simulink model "que2"  (R2023a)
settings: Solver=VariableStepAuto  StartTime=0.0  StopTime=500  RelTol=1e-3
settings Model: Creator=Hasee  LastModifiedBy=Administrator

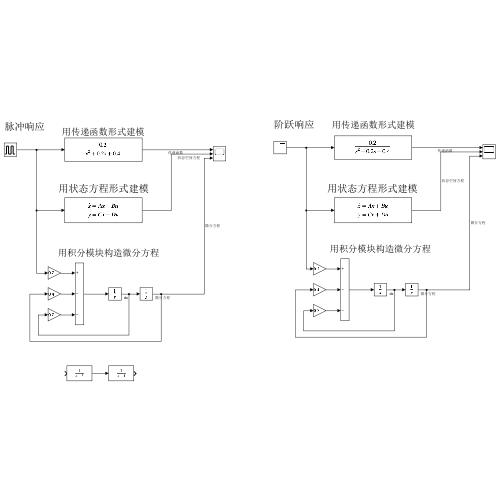
[thumbnail: Simulink's stored preview of the top-level diagram]
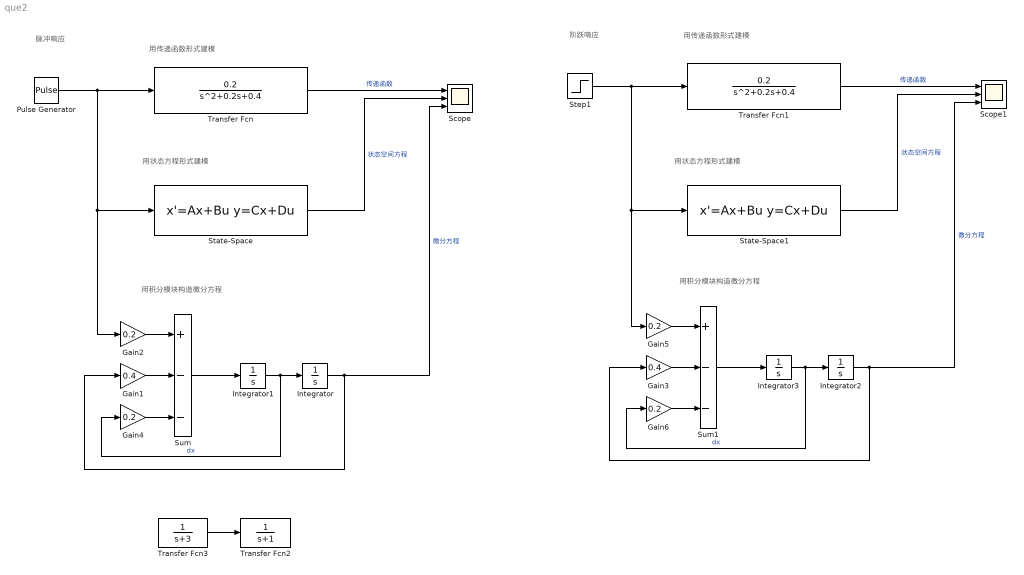
== system que2 ==
  note: 用传递函数形式建模
  note: 用状态方程形式建模
  note: 用积分模块构造微分方程
  note: 脉冲响应
  note: 阶跃响应
  note: 用传递函数形式建模
  note: 用状态方程形式建模
  note: 用积分模块构造微分方程
  Gain1 : Gain  Gain=0.4
  Gain{2,4..6} (4 alike) : Gain  Gain=0.2
  Gain3 : Gain  Gain=0.4
  Integrator{,1..3} (4 alike) : Integrator
  Pulse Generator : DiscretePulseGenerator  PulseType=Time based  Period=150  PulseWidth=55
  Scope : Scope  NumInputPorts=3
  Scope1 : Scope  NumInputPorts=3
  State-Space : StateSpace  A=[0 1;-0.4 -0.2]  B=[0 1]'  C=[0.2 0]  D=0  InitialCondition=0
  State-Space1 : StateSpace  A=[0 1;-0.4 -0.2]  B=[0 1]'  C=[0.2 0]  D=0  InitialCondition=0
  Step1 : Step  SampleTime=0
  Sum : Sum  Inputs=+--
  Sum1 : Sum  Inputs=+--
  Transfer Fcn : TransferFcn  Numerator=[0.2]  Denominator=[1 0.2 0.4]
  Transfer Fcn1 : TransferFcn  Numerator=[0.2]  Denominator=[1 0.2 0.4]
  Transfer Fcn2 : TransferFcn  Denominator=[1 1]
  Transfer Fcn3 : TransferFcn  Denominator=[1 3]
  wires:
  Pulse Generator/1 -> State-Space/1, Gain2/1, Transfer Fcn/1
  Transfer Fcn/1 -> Scope/1  "传递函数"
  State-Space/1 -> Scope/2  "状态空间方程"
  Integrator1/1 -> Gain4/1, Integrator/1  "dx"
  Gain2/1 -> Sum/1
  Gain1/1 -> Sum/2
  Gain4/1 -> Sum/3
  Integrator/1 -> Scope/3, Gain1/1  "微分方程"
  Sum/1 -> Integrator1/1
  Gain3/1 -> Sum1/2
  Integrator2/1 -> Scope1/3, Gain3/1  "微分方程"
  Gain6/1 -> Sum1/3
  Step1/1 -> Gain5/1, State-Space1/1, Transfer Fcn1/1
  Sum1/1 -> Integrator3/1
  State-Space1/1 -> Scope1/2  "状态空间方程"
  Integrator3/1 -> Gain6/1, Integrator2/1  "dx"
  Transfer Fcn1/1 -> Scope1/1  "传递函数"
  Gain5/1 -> Sum1/1
  Transfer Fcn3/1 -> Transfer Fcn2/1
